simulink model "pendulum"  (R2017b)
settings: Solver=VariableStepAuto  StartTime=0.0  StopTime=100  FixedStep=1  RelTol=1e-3
libraries: vrlib x2
settings Model: Creator=squirrel  LastModifiedBy=squirrel

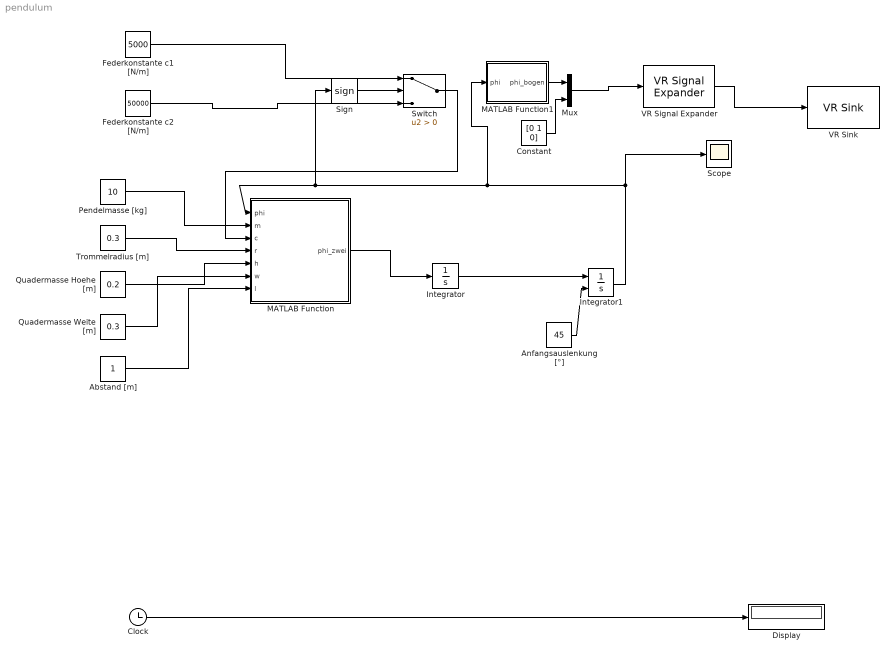
== system pendulum ==
  Abstand [m] : Constant
  Anfangsauslenkung [°] : Constant  Value=45
  Clock : Clock
  Constant : Constant  Value=[0 1 0]
  Display : Display
  Federkonstante c1 [N/m] : Constant  Value=5000
  Federkonstante c2 [N/m] : Constant  Value=50000
  Integrator : Integrator
  Integrator1 : Integrator  InitialConditionSource=external  InitialCondition=45
  MATLAB Function : MATLAB Function  TreatAsAtomicUnit=on
  MATLAB Function1 : MATLAB Function  TreatAsAtomicUnit=on
  Mux : Mux  Inputs=2
  Pendelmasse [kg] : Constant  Value=10
  Quadermasse Hoehe [m] : Constant  Value=0.2
  Quadermasse Weite [m] : Constant  Value=0.3
  Scope : Scope
  Sign : Signum
  Switch : Switch  Criteria=u2 > Threshold
  Trommelradius [m] : Constant  Value=0.3
  VR Signal Expander : vrlib/VR Signal Expander  outwidth=4  outidx=[4 1 2 3]
      settings: SourceProductName=Simulink 3D Animation  SourceProductBaseCode=VR
  VR Sink : vrlib/VR Sink  InstantiateOnLoad=on  SampleTime=0.005  ViewEnable=on  RemoteChange=off  RemoteView=off  FieldsWritten=Seiltrommel.rotation.4.1.1.double  WorldFileName=CrazyPendlm.wrl  AutoView=off  VideoDimensions=[]  AllowVariableSize=off
      settings: SourceProductBaseCode=VR
  wires:
  Abstand [m]/1 -> MATLAB Function/7(l)
  Quadermasse Weite [m]/1 -> MATLAB Function/6(w)
  Quadermasse Hoehe [m]/1 -> MATLAB Function/5(h)
  Trommelradius [m]/1 -> MATLAB Function/4(r)
  Pendelmasse [kg]/1 -> MATLAB Function/2(m)
  Anfangsauslenkung [°]/1 -> Integrator1/2
  Integrator/1 -> Integrator1/1
  MATLAB Function/1(phi_zwei) -> Integrator/1
  Integrator1/1 -> Scope/1, MATLAB Function1/1(phi), Sign/1, MATLAB Function/1(phi)
  Federkonstante c1 [N/m]/1 -> Switch/1
  Federkonstante c2 [N/m]/1 -> Switch/3
  Switch/1 -> MATLAB Function/3(c)
  Clock/1 -> Display/1
  Sign/1 -> Switch/2
  VR Signal Expander/1 -> VR Sink/1
  Constant/1 -> Mux/2
  Mux/1 -> VR Signal Expander/1
  MATLAB Function1/1(phi_bogen) -> Mux/1

== matlab function pendulum/MATLAB Function1 ==
  data: phi input; phi_bogen output
function phi_bogen = fcn(phi)

phi_bogen = (phi / 180) * pi;

== matlab function pendulum/MATLAB Function ==
  data: phi input; phi_zwei output; m input; c input; r input; h input; w input; l input
function phi_zwei = winkelgeschw(phi, m, c, r, h, w, l)

g = 9.81;

%phi_bogen = (phi / 180) * pi; % phi in Bogenmass [Radien]
%J = (1/12) * m * (w^2 * h^2) + m * (l + (h/2))^2;
%F = -c * phi_bogen * r^2 + m * g * sin(phi_bogen) * (l + (h/2))^2;
%phi_zwei = F / J;


if phi < 90
    wbog = phi * pi/180;   
    
    rP1 = l+r+0.5*h;
    rP2 = sin(wbog)*rP1;
    
    fF1 = -c * wbog * r^2;
    fP1 = (m * g / tan(wbog)) * rP2;
    J = 0.5*m * r^2;
    phi_zwei = (fF1 + fP1) / J;
    
    
else
    if phi == 90
        phi_zwei = 0;
    else 
        
        wbog = (phi - 90) * pi / 180;
       % w2bog = (180 - winkel) * pi / 180;
        
        
        rP1 = l+r+0.5*h;
        rP2 = sin(wbog)*rP1;

        fF2 = c * wbog * r^2;
        fP2 = -(m * g * tan(wbog)) * rP2;
        J = 0.5*m * r^2;
        phi_zwei = (fF2 + fP2) / J;
        
        %f1 = -(pendelMasse * g * tan(wbog) * (0.5*h + l + r));
        %f2 = (c2 * w2bog *r^2);
        %J = 1 / ((1/12) *pendelMasse * (a^2 + h^2) + pendelMasse * (l/2)^2);
        %winkelgeschw =  (f1+f2)*J;
    end
        
end




% phi = Winkel des Pendels [°]; m = Pendelmasse [kg]; c = Federkonstante der aktiven Feder [N/m]; r =
% Seiltrommelradius [m]; h = Hoehe Quadermasse [m]; w = Weite Quadermasse [m]; l =
% Laenge Pendelstange [m]
%g = -9.81; % Schwerkraft [m/s^2]
%G = m * g; % Gravitationskraft [N]
%phi_bogen = (phi / 180) * pi; % phi in Bogenmass [Radien]
%weg = phi_bogen * r; % Umfang der Umdrehung der Pendeltrommel [m]
%F_g1 = G / cos(phi_bogen); % Zugkraft durch Gravitation [N]
%F_z1 = -c * weg; % aeussere Zugkraft [N]

%F_x1 = c * -(weg);
%F_x2 = -c * weg;
%F_y1 = sin(phi_bogen) * F_x1;
%F_y2 = sin(phi_bogen) * F_x2;
%massetraegheit = ((m / 12) * (h^2 + w^2)) + m * ((h / 2) + l + r)^2;

%phi_zwei = (((F_g1 + F_z1) * r) / massetraegheit) * (180 / pi);
%phi_zwei = (((F_x1 + F_x2) * r) / massetraegheit) * r;
